simulink model "Projet_Modele_Interne_sim_LIMA_MILITAO_PINHEIRO"  (R2019a)
settings: Solver=VariableStepAuto  StartTime=0.0  StopTime=10.0  FixedStep=1e-6  RelTol=1e-3
undefined symbols (not defined in the file): Am_omega, Bm_omega, Cz_den_MI, Cz_num_MI, den, F_den_MI, F_num_MI, G2d_den, G2d_num, G_den_MI, G_num_MI, numG2, Te, tsim
settings Model: Creator=dougl  LastModifiedBy=dougl
settings DebuggingCC: UnconnectedInputMsg=none  UnconnectedOutputMsg=none  UnconnectedLineMsg=none  SFMachineParentedDataDiag=error

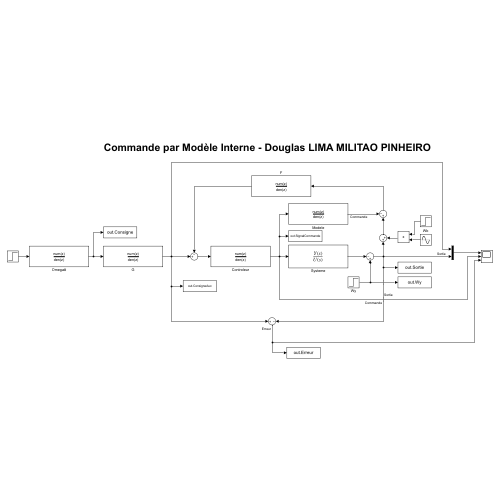
[thumbnail: Simulink's stored preview of the top-level diagram]
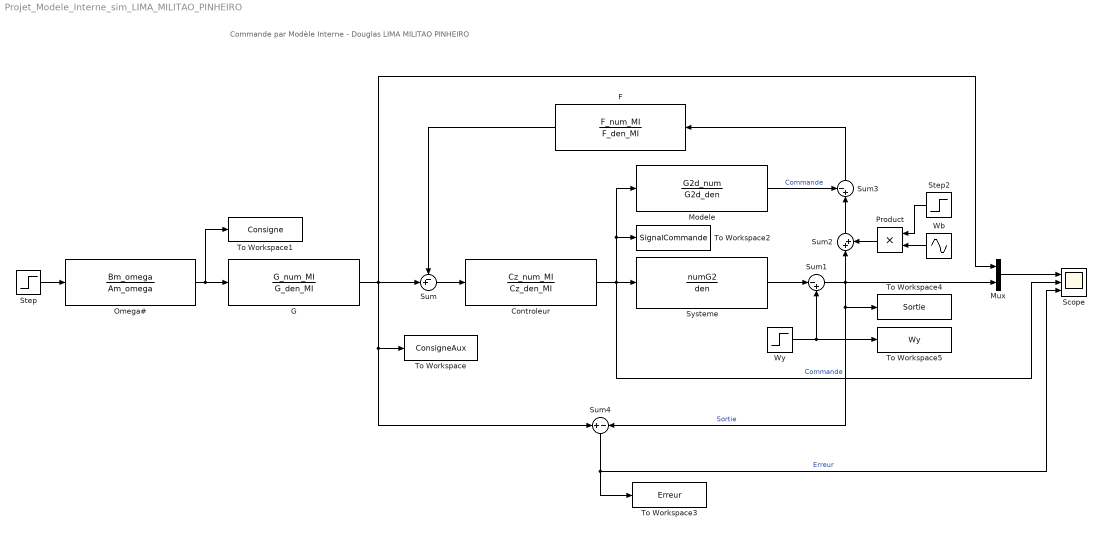
== system Projet_Modele_Interne_sim_LIMA_MILITAO_PINHEIRO ==
  note: Commande par Modèle Interne - Douglas LIMA MILITAO PINHEIRO
  Controleur : DiscreteFilter  Numerator=Cz_num_MI  Denominator=Cz_den_MI  SampleTime=Te
  F : DiscreteFilter  Numerator=F_num_MI  Denominator=F_den_MI  SampleTime=Te
  G : DiscreteFilter  Numerator=G_num_MI  Denominator=G_den_MI  SampleTime=Te
  Modele : DiscreteFilter  Numerator=G2d_num  Denominator=G2d_den  SampleTime=Te
  Mux : Mux  Inputs=2
  Omega# : DiscreteFilter  Numerator=Bm_omega  Denominator=Am_omega  SampleTime=Te
  Product : Product
  Scope : Scope  NumInputPorts=3
  Step : Step  After=5  SampleTime=0
  Step2 : Step  Time=7  SampleTime=0
  Sum : Sum  Inputs=-+|
  Sum1 : Sum  Inputs=|-+
  Sum2 : Sum  Inputs=|++
  Sum3 : Sum  Inputs=-+|
  Sum4 : Sum  Inputs=+|-
  Systeme : TransferFcn  Numerator=numG2  Denominator=den
  To Workspace : ToWorkspace  VariableName=ConsigneAux  SampleTime=tsim
  To Workspace1 : ToWorkspace  VariableName=Consigne  SampleTime=tsim
  To Workspace2 : ToWorkspace  VariableName=SignalCommande  SampleTime=tsim
  To Workspace3 : ToWorkspace  VariableName=Erreur  SampleTime=tsim
  To Workspace4 : ToWorkspace  VariableName=Sortie  SampleTime=tsim
  To Workspace5 : ToWorkspace  VariableName=Wy  SampleTime=tsim
  Wb : Sin  Amplitude=3  Frequency=2*pi*10  SampleTime=0
  Wy : Step  Time=5  After=15  SampleTime=0
  wires:
  Sum/1 -> Controleur/1
  Step/1 -> Omega#/1
  Systeme/1 -> Sum1/1
  Wy/1 -> Sum1/2, To Workspace5/1
  Controleur/1 -> Modele/1, To Workspace2/1, Scope/2, Systeme/1  "Commande"
  Mux/1 -> Scope/1
  Modele/1 -> Sum3/1  "Commande"
  F/1 -> Sum/1
  Sum3/1 -> F/1
  Step2/1 -> Product/1
  Wb/1 -> Product/2
  Product/1 -> Sum2/2
  Sum2/1 -> Sum3/2
  Omega#/1 -> G/1, To Workspace1/1
  G/1 -> Mux/1, Sum/2, Sum4/1, To Workspace/1
  Sum4/1 -> To Workspace3/1, Scope/3  "Erreur"
  Sum1/1 -> Mux/2, Sum2/1, To Workspace4/1, Sum4/2  "Sortie"
